simulink model "BicycleSimulation"  (R2020a)
settings: Solver=FixedStepAuto  StartTime=0.0  StopTime=inf  FixedStep=0.005  RelTol=1e-3  EnableMultiTasking=on
libraries: simulink x11
settings Model: NumberOfSteps=2  EnablePacing=on  Creator=Admin  LastModifiedBy=Robin Vogt
settings DataIOCC: ReturnWorkspaceOutputs=off
settings OptimizationCC: LifeSpan=inf
settings DebuggingCC: SFUnexpectedBacktrackingDiag=warning  SFNoUnconditionalDefaultTransitionDiag=warning  SFExecutionAtInitializationDiag=none  UnderSpecifiedDimensionMsg=warning  ArithmeticOperatorsInVariantConditions=warning
settings SFSimCC: SimUseLocalCustomCode=off  CustomCodeUndefinedFunction=UseInterfaceOnly
settings RTWCC: RTWUseLocalCustomCode=off
settings CodeAppCC: StateflowObjectComments=on
settings GRTTargetCC: TargetLangStandard=C89/C90 (ANSI)
settings ConfigComp: CovMetricSettings=dw  CovHtmlReporting=on  CovSaveCumulativeToWorkspaceVar=on  CovSaveSingleToWorkspaceVar=on  CovExternalEMLEnable=off

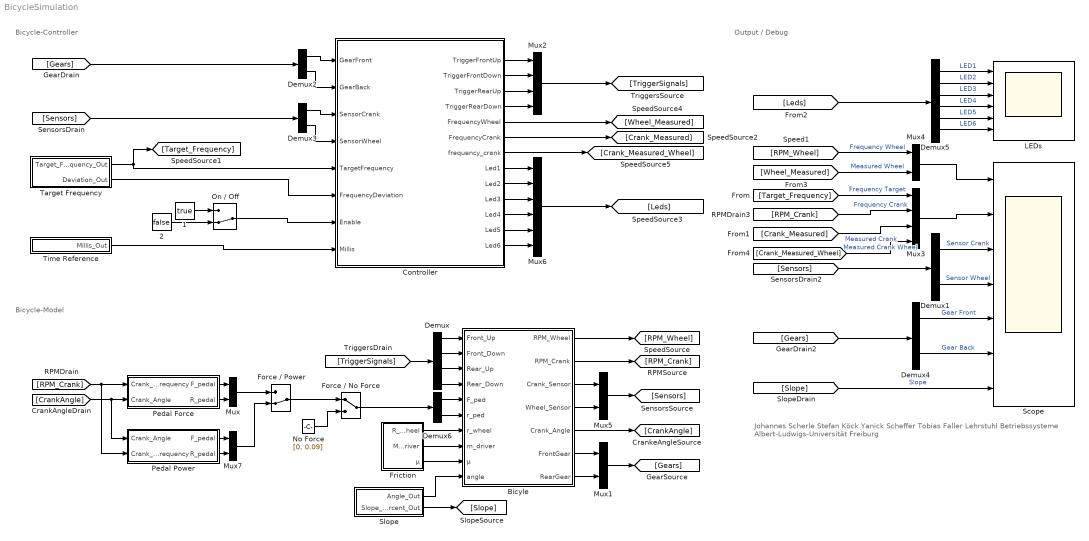
== system BicycleSimulation ==
  note: Bicycle-Model
  note: Johannes Scherle
      | Stefan Köck
      | Yanick Scheffer
      | Tobias Faller
      | Lehrstuhl Betriebssysteme
      | Albert-Ludwigs-Universität Freiburg
  note: Bicycle-Controller
  note: Output / Debug
  1 : Constant  Value=true  OutDataTypeStr=boolean
  2 : Constant  Value=false  OutDataTypeStr=boolean
  Bicyle : Subsystem
  Controller : Stateflow chart  TreatAsAtomicUnit=on  SystemSampleTime=0.005
      settings: PortSchema="{\"entries\":[{\"content\":{\"sides\":[{\"content\":{\"connectorIds\":[\"In1\",\"In2\",\"In3\",\"In4\",\"In5\",\"In6\",\"In7\",\"In8\"]},\"type\":\"ConnectorPlacement.EquallySpacedRectSide\",\"uuid\":\"1754ec92-7cce-411a-82a3-2fbca3fb4c28\"},{\"content\":{\"connectorIds\":[\"Out1\",\"Out2\",\"Out3\",\"Out4\",\"Out5\",\"Out6\",\"Out13\",\"Out7\",\"Out8\",\"Out9\",\"Out10\",\"Out11\",\"Out12\"],\"side\":\"RIGHT\"},\"type\":\"ConnectorPlacement.EquallySpacedRectSide\",\"uuid\":\"9c6a9c26-d673-4feb-91f9-24c7e2d76c42\"},{\"content\":{\"connectorIds\":[],\"side\":\"TOP\"},\"type\":\"ConnectorPlacement.EquallySpacedRectSide\",\"uuid\":\"a2f456d0-fed3-444f-af5e-51a24e4e3fa9\"}]},\"type\":\"ConnectorPlacement.EquallySpacedConnector\",\"uuid\":\"42155252-21b8-44f1-bf8e-e9314f1d83ec\"}],\"packageUris\":[\"http://schema.mathworks.com/mf0/Connector/19700101\"],\"version\":\"1.0\"}"
  Demux : Demux
  Demux{1..4,6} (5 alike) : Demux  Outputs=2
  Demux5 : Demux  Outputs=6
  Force / No Force : ManualSwitch
  Force / Power : ManualSwitch  CurrentSetting=0
  Friction : Subsystem
  LEDs : Scope  NumInputPorts=6
  Mux{,1,5,7} (4 alike) : Mux  Inputs=2
  Mux2 : Mux
  Mux3 : Mux  Inputs=Frequency Target,Frequency Crank,Measured Crank,Measured Crank Wheel
  Mux4 : Mux  Inputs=Frequency Wheel,Measured Wheel
  Mux6 : Mux  Inputs=6
  No Force : Constant  Value=[0, 0.09]  VectorParams1D=off  OutDataTypeStr=double
  On / Off : ManualSwitch  CurrentSetting=0
  Pedal Force : Subsystem
  Pedal Power : Subsystem
  Scope : Scope  NumInputPorts=7
  Slope : Subsystem
  Target Frequency : Subsystem
  Time Reference : Subsystem
  wires:
  Slope/1(Angle_Out) -> Bicyle/10(angle)
  Target Frequency/1(Target_Frequency_Out) -> Controller/5(TargetFrequency), [Target_Frequency]
  Target Frequency/2(Deviation_Out) -> Controller/6(FrequencyDeviation)
  Time Reference/1(Millis_Out) -> Controller/8(Millis)
  Bicyle/3(Crank_Sensor) -> Mux5/1
  Bicyle/4(Wheel_Sensor) -> Mux5/2
  Bicyle/6(FrontGear) -> Mux1/1
  Bicyle/7(RearGear) -> Mux1/2
  Controller/2(TriggerFrontDown) -> Mux2/2
  Controller/3(TriggerRearUp) -> Mux2/3
  Controller/1(TriggerFrontUp) -> Mux2/1
  Controller/4(TriggerRearDown) -> Mux2/4
  Demux/1 -> Bicyle/1(Front_Up)
  Demux/2 -> Bicyle/2(Front_Down)
  Demux/3 -> Bicyle/3(Rear_Up)
  Demux/4 -> Bicyle/4(Rear_Down)
  Mux2/1 -> [TriggerSignals]
  Demux4/1 -> Scope/5  "Gear Front"
  Demux4/2 -> Scope/6  "Gear Back"
  [TriggerSignals] -> Demux/1
  [Gears] -> Demux4/1
  Demux2/1 -> Controller/1(GearFront)
  Demux2/2 -> Controller/2(GearBack)
  Mux1/1 -> [Gears]
  Mux5/1 -> [Sensors]
  Friction/3(µ) -> Bicyle/9(µ)
  Friction/2(M_Driver) -> Bicyle/8(m_driver)
  Friction/1(R_Wheel) -> Bicyle/7(r_wheel)
  Demux1/2 -> Scope/4  "Sensor Wheel"
  [Sensors] -> Demux1/1
  Demux3/1 -> Controller/3(SensorCrank)
  Demux3/2 -> Controller/4(SensorWheel)
  Slope/2(Slope_Percent_Out) -> [Slope]
  [Slope] -> Scope/7  "Slope"
  Bicyle/5(Crank_Angle) -> [CrankAngle]
  [CrankAngle] -> Pedal Power/1(Crank_Angle), Pedal Force/2(Crank_Angle)
  Demux1/1 -> Scope/3  "Sensor Crank"
  Mux3/1 -> Scope/2
  Bicyle/2(RPM_Crank) -> [RPM_Crank]
  [RPM_Crank] -> Pedal Power/2(Crank_Frequency), Pedal Force/1(Crank_Frequency)
  [RPM_Crank] -> Mux3/2  "Frequency Crank"
  [Target_Frequency] -> Mux3/1  "Frequency Target"
  [Crank_Measured] -> Mux3/3  "Measured Crank"
  Controller/7(Led1) -> Mux6/1
  Controller/8(Led2) -> Mux6/2
  Controller/9(Led3) -> Mux6/3
  Controller/10(Led4) -> Mux6/4
  Controller/11(Led5) -> Mux6/5
  Controller/12(Led6) -> Mux6/6
  On / Off/1 -> Controller/7(Enable)
  1/1 -> On / Off/1
  2/1 -> On / Off/2
  Mux6/1 -> [Leds]
  [Sensors] -> Demux3/1
  [Gears] -> Demux2/1
  [Leds] -> Demux5/1
  Demux5/1 -> LEDs/1  "LED1"
  Demux5/2 -> LEDs/2  "LED2"
  Demux5/3 -> LEDs/3  "LED3"
  Demux5/4 -> LEDs/4  "LED4"
  Demux5/5 -> LEDs/5  "LED5"
  Demux5/6 -> LEDs/6  "LED6"
  Controller/5(FrequencyWheel) -> [Wheel_Measured]
  Bicyle/1(RPM_Wheel) -> [RPM_Wheel]
  Mux4/1 -> Scope/1
  [Wheel_Measured] -> Mux4/2  "Measured Wheel"
  [RPM_Wheel] -> Mux4/1  "Frequency Wheel"
  Mux/1 -> Force / Power/1
  Mux7/1 -> Force / Power/2
  Demux6/1 -> Bicyle/5(F_ped)
  Demux6/2 -> Bicyle/6(r_ped)
  Force / No Force/1 -> Demux6/1
  Force / Power/1 -> Force / No Force/1
  No Force/1 -> Force / No Force/2
  Pedal Force/1(F_pedal) -> Mux/1
  Pedal Force/2(R_pedal) -> Mux/2
  Pedal Power/1(F_pedal) -> Mux7/1
  Pedal Power/2(R_pedal) -> Mux7/2
  Controller/6(FrequencyCrank) -> [Crank_Measured]
  Controller/13(frequency_crank) -> [Crank_Measured_Wheel]
  [Crank_Measured_Wheel] -> Mux3/4  "Measured Crank Wheel"

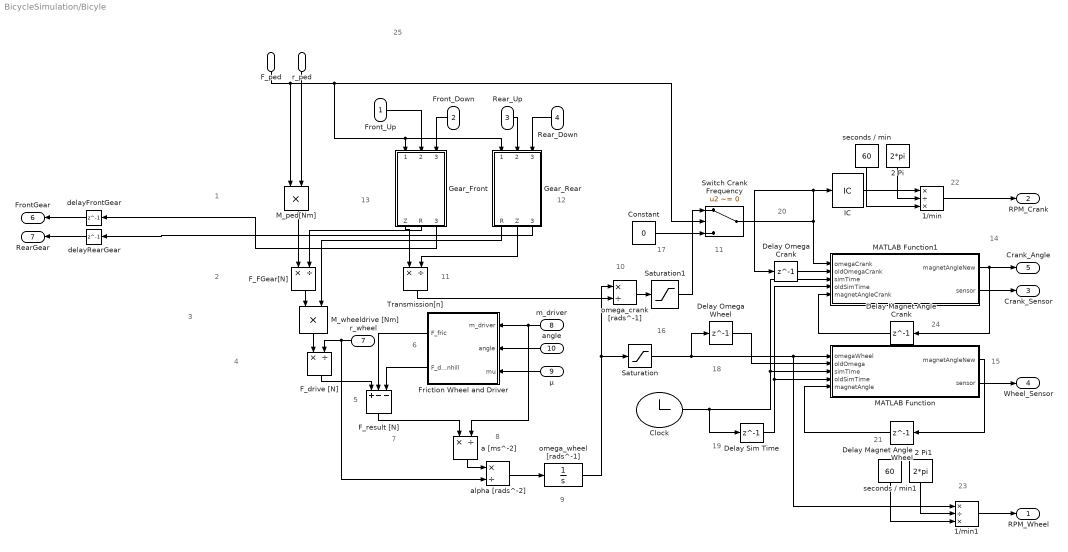
== system BicycleSimulation/Bicyle ==
  note: 1
  note: 2
  note: 3
  note: 4
  note: 5
  note: 6
  note: 7
  note: 8
  note: 9
  note: 10
  note: 11
  note: 11
  note: 12
  note: 13
  note: 14
  note: 15
  note: 16
  note: 17
  note: 18
  note: 19
  note: 20
  note: 21
  note: 22
  note: 23
  note: 24
  note: 25
  Front_Up : Inport
  Front_Down : Inport  Port=2
  Rear_Up : Inport  Port=3
  Rear_Down : Inport  Port=4
  F_ped : Inport  Port=5
  r_ped : Inport  Port=6
  r_wheel : Inport  Port=7
  m_driver : Inport  Port=8
  µ : Inport  Port=9
  angle : Inport  Port=10
  1/min : Product  Inputs=*/*  OutDataTypeStr=double
  1/min1 : Product  Inputs=*/*
  2 Pi : Constant  Value=2*pi
  2 Pi1 : Constant  Value=2*pi
  Clock : Clock
  Constant : Constant  Value=0
  Delay Omega Crank : Delay  DelayLength=1  InitialCondition=1
  Delay Omega Wheel : Delay  DelayLength=1  InitialCondition=0
  Delay Sim Time : Delay  DelayLength=1  InitialCondition=0
  "Delay Magnet Angle Crank " : Delay  DelayLength=1  InitialCondition=0
  Delay Magnet Angle Wheel : Delay  DelayLength=1  InitialCondition=0
  F_FGear[N] : Product  Inputs=*/
  F_drive [N] : Product  Inputs=*/
  F_result [N] : Sum  Inputs=+--
  Friction Wheel and Driver : Subsystem
  Gear_Front : Subsystem
  Gear_Rear : Subsystem
  IC : InitialCondition  Value=0
  MATLAB Function : MATLAB Function  TreatAsAtomicUnit=on
  MATLAB Function1 : MATLAB Function  TreatAsAtomicUnit=on
  M_ped[Nm] : Product
  M_wheeldrive [Nm] : Product
  Saturation : Saturate  UpperLimit=100  LowerLimit=0
  Saturation1 : Saturate  UpperLimit=18  LowerLimit=0
  Switch Crank Frequency : Switch  Criteria=u2 ~= 0
  Transmission[n] : Product  Inputs=*/
  a [ms^-2] : Product  Inputs=*/
  alpha [rads^-2] : Product  Inputs=*/
  delayFrontGear : Delay  DelayLength=1  InitialCondition=0
  delayRearGear : Delay  DelayLength=1  InitialCondition=0
  omega_crank [rads^-1] : Product  Inputs=*/
  omega_wheel [rads^-1] : Integrator  LimitOutput=on  UpperSaturationLimit=60  LowerSaturationLimit=0
  seconds / min : Constant  Value=60
  seconds / min1 : Constant  Value=60
  RPM_Wheel : Outport  VectorParamsAs1DForOutWhenUnconnected=off
  RPM_Crank : Outport  Port=2  VectorParamsAs1DForOutWhenUnconnected=off
  Crank_Sensor : Outport  Port=3  VectorParamsAs1DForOutWhenUnconnected=off
  Wheel_Sensor : Outport  Port=4  VectorParamsAs1DForOutWhenUnconnected=off
  Crank_Angle : Outport  Port=5  VectorParamsAs1DForOutWhenUnconnected=off
  FrontGear : Outport  Port=6  VectorParamsAs1DForOutWhenUnconnected=off
  RearGear : Outport  Port=7  VectorParamsAs1DForOutWhenUnconnected=off
  wires:
  Front_Up/1 -> Gear_Front/2(Trigger_Up)
  Rear_Up/1 -> Gear_Rear/2(Trigger_Up)
  Front_Down/1 -> Gear_Front/3(Trigger_Down)
  F_ped/1 -> Gear_Rear/1(F_ped), Gear_Front/1(F_ped), Switch Crank Frequency/2, M_ped[Nm]/1
  r_ped/1 -> M_ped[Nm]/2
  a [ms^-2]/1 -> alpha [rads^-2]/1
  M_ped[Nm]/1 -> F_FGear[N]/1
  M_wheeldrive [Nm]/1 -> F_drive [N]/1
  F_result [N]/1 -> a [ms^-2]/1
  Gear_Front/1(Z) -> Transmission[n]/1
  Gear_Front/2(R) -> F_FGear[N]/2
  F_FGear[N]/1 -> M_wheeldrive [Nm]/1
  Gear_Rear/1(R) -> M_wheeldrive [Nm]/2
  omega_crank [rads^-1]/1 -> Saturation1/1
  Friction Wheel and Driver/1(F_fric) -> F_result [N]/2
  Clock/1 -> Delay Sim Time/1, MATLAB Function/3(simTime), MATLAB Function1/3(simTime)
  Delay Omega Wheel/1 -> MATLAB Function/2(oldOmega)
  Delay Sim Time/1 -> MATLAB Function1/4(oldSimTime), MATLAB Function/4(oldSimTime)
  MATLAB Function/1(magnetAngleNew) -> Delay Magnet Angle Wheel/1
  Delay Magnet Angle Wheel/1 -> MATLAB Function/5(magnetAngle)
  MATLAB Function/2(sensor) -> Wheel_Sensor/1
  Rear_Down/1 -> Gear_Rear/3(Trigger_Down)
  r_wheel/1 -> F_drive [N]/2, alpha [rads^-2]/2
  F_drive [N]/1 -> F_result [N]/1
  Friction Wheel and Driver/2(F_downhill) -> F_result [N]/3
  m_driver/1 -> a [ms^-2]/2, Friction Wheel and Driver/1(m_driver)
  angle/1 -> Friction Wheel and Driver/2(angle)
  µ/1 -> Friction Wheel and Driver/3(mu)
  alpha [rads^-2]/1 -> omega_wheel [rads^-1]/1
  Gear_Rear/2(Z) -> Transmission[n]/2
  Delay Omega Crank/1 -> MATLAB Function1/2(oldOmegaCrank)
  MATLAB Function1/1(magnetAngleNew) -> "Delay Magnet Angle Crank "/1, Crank_Angle/1
  "Delay Magnet Angle Crank "/1 -> MATLAB Function1/5(magnetAngleCrank)
  MATLAB Function1/2(sensor) -> Crank_Sensor/1
  2 Pi/1 -> 1/min/2
  seconds / min/1 -> 1/min/3
  1/min/1 -> RPM_Crank/1
  Transmission[n]/1 -> omega_crank [rads^-1]/2
  Saturation/1 -> MATLAB Function/1(omegaWheel), 1/min1/1, Delay Omega Wheel/1
  2 Pi1/1 -> 1/min1/2
  seconds / min1/1 -> 1/min1/3
  1/min1/1 -> RPM_Wheel/1
  Switch Crank Frequency/1 -> Delay Omega Crank/1, IC/1, MATLAB Function1/1(omegaCrank)
  IC/1 -> 1/min/1
  omega_wheel [rads^-1]/1 -> omega_crank [rads^-1]/1, Saturation/1
  Gear_Rear/3(gearR) -> delayRearGear/1
  Gear_Front/3(gearF) -> delayFrontGear/1
  delayRearGear/1 -> RearGear/1
  delayFrontGear/1 -> FrontGear/1
  Saturation1/1 -> Switch Crank Frequency/1
  Constant/1 -> Switch Crank Frequency/3

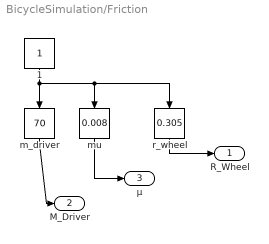
== system BicycleSimulation/Friction ==
  1 : Constant
  m_driver : simulink/Math Operations/Slider Gain  gain=70  low=0  high=150
  mu : simulink/Math Operations/Slider Gain  gain=0.008  low=0  high=0.1
  r_wheel : simulink/Math Operations/Slider Gain  gain=0.305  low=0  high=1
  R_Wheel : Outport  VectorParamsAs1DForOutWhenUnconnected=off
  M_Driver : Outport  Port=2  VectorParamsAs1DForOutWhenUnconnected=off
  µ : Outport  Port=3  VectorParamsAs1DForOutWhenUnconnected=off
  wires:
  m_driver/1 -> M_Driver/1
  r_wheel/1 -> R_Wheel/1
  1/1 -> m_driver/1, r_wheel/1, mu/1
  mu/1 -> µ/1

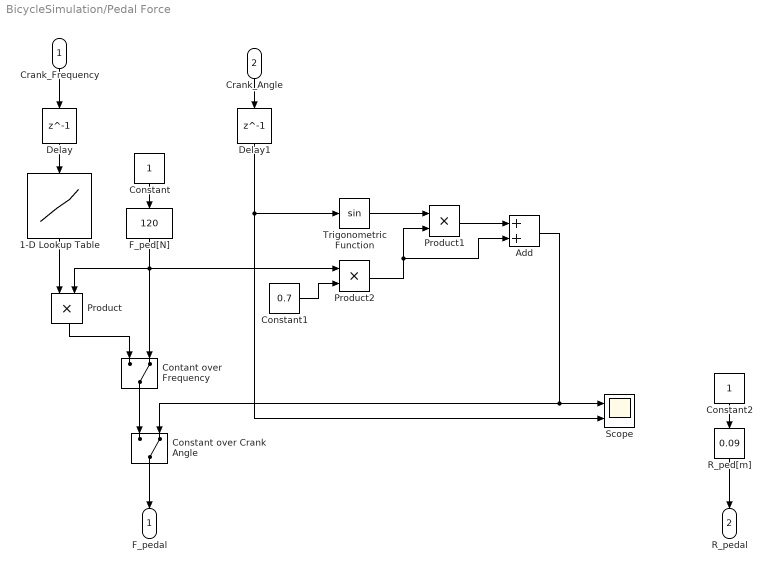
== system BicycleSimulation/Pedal Force ==
  Crank_Frequency : Inport
  Crank_Angle : Inport  Port=2
  1-D Lookup Table : Lookup_n-D  NumberOfTableDimensions=1  BreakpointsForDimension1=[0 10 20 30 40 50 60 70 80 90 100 110 120 130 140 150 160]  Table=[1 1 1 1 1 1 1 1 1 0.99 0.95 0.8 0.7 0.6 0.5 0.3 0]  RndMeth=Simplest  InputSameDT=on
  Add : Sum
  Constant : Constant
  Constant over Crank Angle : ManualSwitch  CurrentSetting=0
  Constant1 : Constant  Value=0.7
  Constant2 : Constant
  Contant over Frequency : ManualSwitch  CurrentSetting=0
  Delay : Delay  DelayLength=1
  Delay1 : Delay  DelayLength=1
  F_ped[N] : simulink/Math Operations/Slider Gain  gain=120  low=0  high=180
  Product : Product
  Product1 : Product
  Product2 : Product
  R_ped[m] : simulink/Math Operations/Slider Gain  gain=0.09  low=0  high=0.3
  Scope : Scope  NumInputPorts=2
  Trigonometric Function : Trigonometry
  F_pedal : Outport  VectorParamsAs1DForOutWhenUnconnected=off
  R_pedal : Outport  Port=2  VectorParamsAs1DForOutWhenUnconnected=off
  wires:
  R_ped[m]/1 -> R_pedal/1
  Constant/1 -> F_ped[N]/1
  F_ped[N]/1 -> Product/2, Contant over Frequency/2, Product2/1
  Product/1 -> Contant over Frequency/1
  1-D Lookup Table/1 -> Product/1
  Trigonometric Function/1 -> Product1/1
  Product2/1 -> Add/2, Product1/2
  Constant1/1 -> Product2/2
  Product1/1 -> Add/1
  Add/1 -> Scope/1, Constant over Crank Angle/2
  Constant over Crank Angle/1 -> F_pedal/1
  Contant over Frequency/1 -> Constant over Crank Angle/1
  Crank_Frequency/1 -> Delay/1
  Delay/1 -> 1-D Lookup Table/1
  Crank_Angle/1 -> Delay1/1
  Delay1/1 -> Trigonometric Function/1, Scope/2
  Constant2/1 -> R_ped[m]/1

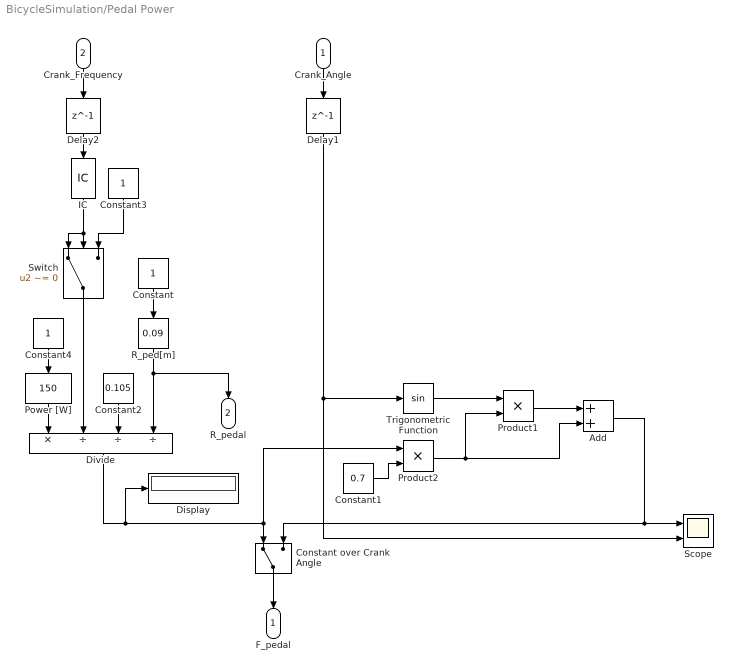
== system BicycleSimulation/Pedal Power ==
  Crank_Angle : Inport
  Crank_Frequency : Inport  Port=2
  Add : Sum
  Constant : Constant
  Constant over Crank Angle : ManualSwitch
  Constant1 : Constant  Value=0.7
  Constant2 : Constant  Value=0.105
  Constant3 : Constant
  Constant4 : Constant
  Delay1 : Delay  DelayLength=1
  Delay2 : Delay  DelayLength=1  InitialCondition=1
  Display : Display
  Divide : Product  Inputs=*///
  IC : InitialCondition
  Power [W] : simulink/Math Operations/Slider Gain  gain=150  low=0  high=200
  Product1 : Product
  Product2 : Product
  R_ped[m] : simulink/Math Operations/Slider Gain  gain=0.09  low=0  high=0.3
  Scope : Scope  NumInputPorts=2
  Switch : Switch  Criteria=u2 ~= 0
  Trigonometric Function : Trigonometry
  F_pedal : Outport  VectorParamsAs1DForOutWhenUnconnected=off
  R_pedal : Outport  Port=2  VectorParamsAs1DForOutWhenUnconnected=off
  wires:
  R_ped[m]/1 -> R_pedal/1, Divide/4
  Constant/1 -> R_ped[m]/1
  Power [W]/1 -> Divide/1
  Trigonometric Function/1 -> Product1/1
  Product2/1 -> Add/2, Product1/2
  Constant1/1 -> Product2/2
  Product1/1 -> Add/1
  Add/1 -> Scope/1, Constant over Crank Angle/2
  Constant over Crank Angle/1 -> F_pedal/1
  Constant2/1 -> Divide/3
  Divide/1 -> Constant over Crank Angle/1, Product2/1, Display/1
  Delay2/1 -> IC/1
  Crank_Frequency/1 -> Delay2/1
  Crank_Angle/1 -> Delay1/1
  Delay1/1 -> Scope/2, Trigonometric Function/1
  IC/1 -> Switch/1, Switch/2
  Constant3/1 -> Switch/3
  Switch/1 -> Divide/2
  Constant4/1 -> Power [W]/1

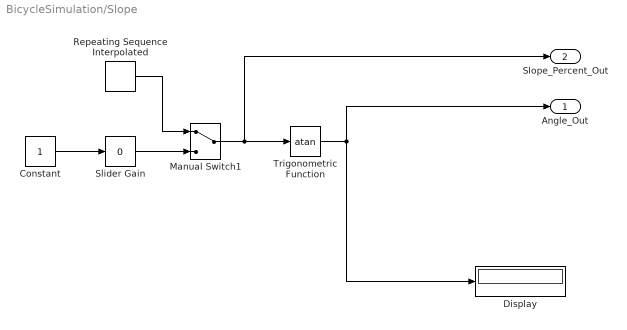
== system BicycleSimulation/Slope ==
  Constant : Constant
  Display : Display
  Manual Switch1 : ManualSwitch
  Repeating Sequence Interpolated : simulink/Sources/Repeating Sequence Interpolated  OutValues=[0 0.01 0.05 0.07 -0.05 -0.01 0].'  TimeValues=[0 2 4 6 8 10 12].'  LookUpMeth=Interpolation-Use End Values  tsamp=0.005  OutMin=[]  OutMax=[]  OutDataTypeStr=double  OutputDataTypeScalingMode=double  OutDataType=fixdt(0,8)  OutScaling=2^-10
  Slider Gain : simulink/Math Operations/Slider Gain  gain=0  low=-1  high=1
  Trigonometric Function : Trigonometry  Operator=atan
  Angle_Out : Outport  VectorParamsAs1DForOutWhenUnconnected=off
  Slope_Percent_Out : Outport  Port=2  VectorParamsAs1DForOutWhenUnconnected=off
  wires:
  Constant/1 -> Slider Gain/1
  Trigonometric Function/1 -> Angle_Out/1, Display/1
  Manual Switch1/1 -> Slope_Percent_Out/1, Trigonometric Function/1
  Slider Gain/1 -> Manual Switch1/2
  Repeating Sequence Interpolated/1 -> Manual Switch1/1

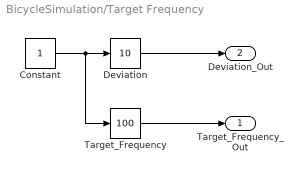
== system BicycleSimulation/Target Frequency ==
  Constant : Constant  OutDataTypeStr=double
  Deviation : simulink/Math Operations/Slider Gain  gain=10  low=0  high=20
  Target_Frequency : simulink/Math Operations/Slider Gain  gain=100  low=0  high=150
  Target_Frequency_Out : Outport  VectorParamsAs1DForOutWhenUnconnected=off
  Deviation_Out : Outport  Port=2  VectorParamsAs1DForOutWhenUnconnected=off
  wires:
  Constant/1 -> Deviation/1, Target_Frequency/1
  Target_Frequency/1 -> Target_Frequency_Out/1
  Deviation/1 -> Deviation_Out/1

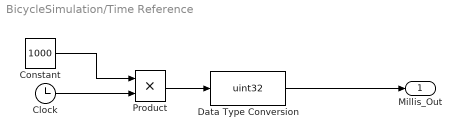
== system BicycleSimulation/Time Reference ==
  Clock : Clock
  Constant : Constant  Value=1000
  Data Type Conversion : DataTypeConversion  OutDataTypeStr=uint32
  Product : Product
  Millis_Out : Outport  SampleTime=0.005  VectorParamsAs1DForOutWhenUnconnected=off
  wires:
  Clock/1 -> Product/2
  Data Type Conversion/1 -> Millis_Out/1
  Product/1 -> Data Type Conversion/1
  Constant/1 -> Product/1

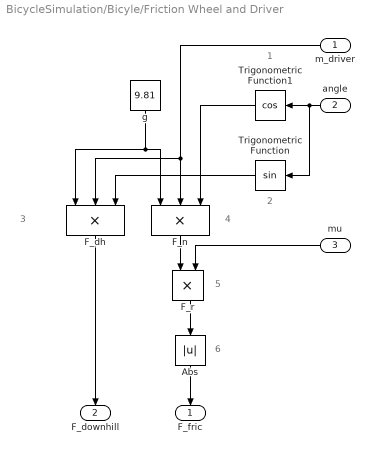
== system BicycleSimulation/Bicyle/Friction Wheel and Driver ==
  note: 1
  note: 2
  note: 3
  note: 4
  note: 5
  note: 6
  m_driver : Inport
  angle : Inport  Port=2
  mu : Inport  Port=3
  Abs : Abs
  F_dh : Product  Inputs=3
  F_n : Product  Inputs=3
  F_r : Product
  Trigonometric Function : Trigonometry
  Trigonometric Function1 : Trigonometry  Operator=cos
  g : Constant  Value=9.81
  F_fric : Outport  VectorParamsAs1DForOutWhenUnconnected=off
  F_downhill : Outport  Port=2  VectorParamsAs1DForOutWhenUnconnected=off
  wires:
  g/1 -> F_dh/1, F_n/1
  Abs/1 -> F_fric/1
  F_n/1 -> F_r/1
  F_r/1 -> Abs/1
  m_driver/1 -> F_dh/2, F_n/2
  Trigonometric Function1/1 -> F_n/3
  mu/1 -> F_r/2
  Trigonometric Function/1 -> F_dh/3
  F_dh/1 -> F_downhill/1
  angle/1 -> Trigonometric Function1/1, Trigonometric Function/1

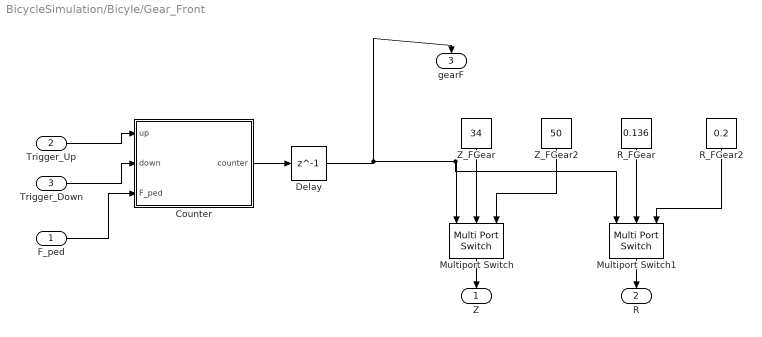
== system BicycleSimulation/Bicyle/Gear_Front ==
  F_ped : Inport
  Trigger_Up : Inport  Port=2
  Trigger_Down : Inport  Port=3
  Counter : Stateflow chart  TreatAsAtomicUnit=on
  Delay : Delay  DelayLength=1
  Multiport Switch : MultiPortSwitch  Inputs=2  DiagnosticForDefault=Warning
  Multiport Switch1 : MultiPortSwitch  Inputs=2  DiagnosticForDefault=Warning
  R_FGear : Constant  Value=0.136
  R_FGear2 : Constant  Value=0.2
  Z_FGear : Constant  Value=34
  Z_FGear2 : Constant  Value=50
  Z : Outport  VectorParamsAs1DForOutWhenUnconnected=off
  R : Outport  Port=2  VectorParamsAs1DForOutWhenUnconnected=off
  gearF : Outport  Port=3  VectorParamsAs1DForOutWhenUnconnected=off
  wires:
  Z_FGear2/1 -> Multiport Switch/3
  Z_FGear/1 -> Multiport Switch/2
  R_FGear/1 -> Multiport Switch1/2
  R_FGear2/1 -> Multiport Switch1/3
  Multiport Switch/1 -> Z/1
  Multiport Switch1/1 -> R/1
  Trigger_Down/1 -> Counter/2(down)
  Trigger_Up/1 -> Counter/1(up)
  F_ped/1 -> Counter/3(F_ped)
  Counter/1(counter) -> Delay/1
  Delay/1 -> Multiport Switch1/1, Multiport Switch/1, gearF/1

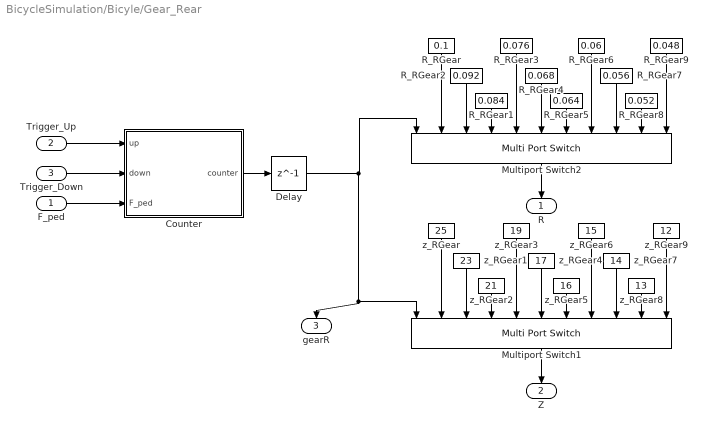
== system BicycleSimulation/Bicyle/Gear_Rear ==
  F_ped : Inport
  Trigger_Up : Inport  Port=2
  Trigger_Down : Inport  Port=3
  Counter : Stateflow chart  TreatAsAtomicUnit=on
  Delay : Delay  DelayLength=1
  Multiport Switch1 : MultiPortSwitch  Inputs=10  DiagnosticForDefault=Warning
  Multiport Switch2 : MultiPortSwitch  Inputs=10  DiagnosticForDefault=Warning
  R_RGear : Constant  Value=0.1
  R_RGear1 : Constant  Value=0.084
  R_RGear2 : Constant  Value=0.092
  R_RGear3 : Constant  Value=0.076
  R_RGear4 : Constant  Value=0.068
  R_RGear5 : Constant  Value=0.064
  R_RGear6 : Constant  Value=0.06
  R_RGear7 : Constant  Value=0.056
  R_RGear8 : Constant  Value=0.052
  R_RGear9 : Constant  Value=0.048
  z_RGear : Constant  Value=25
  z_RGear1 : Constant  Value=23
  z_RGear2 : Constant  Value=21
  z_RGear3 : Constant  Value=19
  z_RGear4 : Constant  Value=17
  z_RGear5 : Constant  Value=16
  z_RGear6 : Constant  Value=15
  z_RGear7 : Constant  Value=14
  z_RGear8 : Constant  Value=13
  z_RGear9 : Constant  Value=12
  R : Outport  VectorParamsAs1DForOutWhenUnconnected=off
  Z : Outport  Port=2  VectorParamsAs1DForOutWhenUnconnected=off
  gearR : Outport  Port=3  VectorParamsAs1DForOutWhenUnconnected=off
  wires:
  R_RGear2/1 -> Multiport Switch2/3
  R_RGear/1 -> Multiport Switch2/2
  Multiport Switch2/1 -> R/1
  Trigger_Down/1 -> Counter/2(down)
  Trigger_Up/1 -> Counter/1(up)
  R_RGear1/1 -> Multiport Switch2/4
  R_RGear3/1 -> Multiport Switch2/5
  R_RGear4/1 -> Multiport Switch2/6
  R_RGear5/1 -> Multiport Switch2/7
  R_RGear8/1 -> Multiport Switch2/10
  R_RGear7/1 -> Multiport Switch2/9
  R_RGear6/1 -> Multiport Switch2/8
  z_RGear1/1 -> Multiport Switch1/3
  z_RGear/1 -> Multiport Switch1/2
  Multiport Switch1/1 -> Z/1
  z_RGear2/1 -> Multiport Switch1/4
  z_RGear3/1 -> Multiport Switch1/5
  z_RGear4/1 -> Multiport Switch1/6
  z_RGear5/1 -> Multiport Switch1/7
  z_RGear8/1 -> Multiport Switch1/10
  z_RGear7/1 -> Multiport Switch1/9
  z_RGear6/1 -> Multiport Switch1/8
  z_RGear9/1 -> Multiport Switch1/11
  R_RGear9/1 -> Multiport Switch2/11
  F_ped/1 -> Counter/3(F_ped)
  Counter/1(counter) -> Delay/1
  Delay/1 -> Multiport Switch1/1, gearR/1, Multiport Switch2/1

== stateflow chart BicycleSimulation/Controller ==
  settings: updateMethod=DISCRETE  sampleTime=0.005
  state Enabled
    state Calculations/ [parallel]
      gear = uint8(6)*(GearFront - uint8(1)) + GearBack;
      settings: executionOrder=1
      state Wheel_Speed_Calculation [parallel]
        settings: executionOrder=1
        state Signal
        Enabled.Calculations.Wheel_Speed_Calculation.Signal -> Enabled.Calculations.Wheel_Speed_Calculation.Signal [order 1] : [Millis >= start_time + time_interval && hasChangedTo(SensorWheel, 0)]/{
            | FrequencyWheel = double(6e4*(sensor_count+1)/(time_interval*16));
            | sensor_count = 0;
            | start_time = Millis;
            | }
        (default) -> Enabled.Calculations.Wheel_Speed_Calculation.Signal
        Enabled.Calculations.Wheel_Speed_Calculation.Signal -> Enabled.Calculations.Wheel_Speed_Calculation.Signal [order 2] : [ Millis < start_time + time_interval && hasChangedTo(SensorWheel, 0)]/{
            | sensor_count = sensor_count +  1;
            | }
      state Force [parallel]
        settings: executionOrder=3
        state Signal/
          en: start_time = Millis;
        Enabled.Calculations.Force.Signal -> Enabled.Calculations.Force.Signal [order 1] : [Millis < start_time + no_force_interval && hasChangedTo(SensorCrank, 0)]/
            | {force = true;}
        (default) -> Enabled.Calculations.Force.Signal
        Enabled.Calculations.Force.Signal -> Enabled.Calculations.Force.Signal [order 2] : [Millis >= start_time + no_force_interval]/{force = false;}
      state Crank_Speed_Calculation [parallel]
        settings: executionOrder=2
        state Signal/
          en: start_time = Millis;
        (default) -> Enabled.Calculations.Crank_Speed_Calculation.Signal
        Enabled.Calculations.Crank_Speed_Calculation.Signal -> Enabled.Calculations.Crank_Speed_Calculation.Signal : [hasChangedTo(SensorCrank, 0)]/{
            | period = Millis-start_time;
            | no_force_interval = 2*period;
            | FrequencyCrank = double(6e4/period);
            | }
    state Shifting [parallel]
      settings: executionOrder=2
      state Shift_gears/
        target_gear_front = idivide(target_gear - uint8(1),  uint8(8)) + uint8(1);
        target_gear_back = target_gear - uint8(6)*(target_gear_front - uint8(1));
        state Rear
          state Up
          state Timer/
            en:
            TriggerRearDown = false;
            TriggerRearUp = false;
            mutex = false;
            start_time = Millis;
            ex:
            mutex = true;
          state Down
          Enabled.Shifting.Shift_gears.Rear.Up -> (junction 210)
          (junction 204) -> Enabled.Shifting.Shift_gears.Rear.Up [order 2] : [GearBack < target_gear_back]/{TriggerRearUp = true;}
          (default) -> Enabled.Shifting.Shift_gears.Rear.Timer
          (junction 210) -> Enabled.Shifting.Shift_gears.Rear.Timer : [Millis >= start_time + uint32(50)]/
              | {servo_timer_rear = Millis;}
          Enabled.Shifting.Shift_gears.Rear.Timer -> (junction 204) : [Millis - servo_timer_rear > uint32(100)]
          Enabled.Shifting.Shift_gears.Rear.Down -> (junction 210)
          (junction 204) -> Enabled.Shifting.Shift_gears.Rear.Down [order 1] : [GearBack > target_gear_back]/{TriggerRearDown = true;}
        state Front
          state Up
          state Timer/
            en:
            TriggerFrontDown = false;
            TriggerFrontUp = false;
            mutex = false;
            start_time = Millis;
            ex:
            mutex = true;
          state Down
          Enabled.Shifting.Shift_gears.Front.Up -> (junction 194)
          (default) -> Enabled.Shifting.Shift_gears.Front.Timer
          (junction 187) -> Enabled.Shifting.Shift_gears.Front.Up [order 1] : [GearFront < target_gear_front]/{TriggerFrontUp = true;}
          Enabled.Shifting.Shift_gears.Front.Timer -> (junction 187) : [Millis - servo_timer_front > 500]
          (junction 194) -> Enabled.Shifting.Shift_gears.Front.Timer : [Millis >= start_time + 600]/
              | {servo_timer_front = Millis;}
          (junction 187) -> Enabled.Shifting.Shift_gears.Front.Down [order 2] : [GearFront > target_gear_front]/{TriggerFrontDown = true;}
          Enabled.Shifting.Shift_gears.Front.Down -> (junction 194)
        Rear -> Front : [GearFront ~= target_gear_front && GearBack > 2 && GearBack < 9]
        (default) -> Rear
        Front -> Rear : [GearFront == target_gear_front]
      state Shifting_decision/
        en:
        translation = translations(gear);
        du:
        frequency_crank = FrequencyWheel/translation;
        state Constant_speed
        state Timer/
          en:
          start_time = Millis;
        state Find_target_gear/
          en:
          lower_bound = bounds(1, index);
          upper_bound = bounds(2, index);
        (default) -> Constant_speed
        Constant_speed -> Enabled.Shifting.Shifting_decision.Timer : [frequency_crank > TargetFrequency + FrequencyDeviation || frequency_crank < TargetFrequency - FrequencyDeviation]
        Enabled.Shifting.Shifting_decision.Timer -> Constant_speed [order 2] : [frequency_crank > TargetFrequency - FrequencyDeviation && frequency_crank < TargetFrequency + FrequencyDeviation]
        (junction 233) -> Constant_speed
        Enabled.Shifting.Shifting_decision.Timer -> Find_target_gear [order 1] : [Millis >= start_time + buffer]/
            | {target_translation = FrequencyWheel/TargetFrequency;
            | index = gear;}
        Find_target_gear -> Find_target_gear [order 3] : [target_translation < lower_bound]/
            | {index = index - 1;}
        Find_target_gear -> Find_target_gear [order 2] : [target_translation > upper_bound]/
            | {index = index + 1;}
        Find_target_gear -> (junction 234) [order 1] : [target_translation <= upper_bound && target_translation >= lower_bound]/
            | {target_gear = index;}
        (junction 234) -> (junction 233)
      state Wait_for_Measurement
      note: need to guard that transition with a mutex
      (default) -> Wait_for_Measurement
      Shifting_decision -> Shift_gears : [gear ~= target_gear && force]
      Wait_for_Measurement -> Shifting_decision : [hasChanged(GearFront) && hasChanged(GearBack)]/
          | {gear = uint8(6)*(GearFront - uint8(1)) + GearBack;}
      Shift_gears -> Shifting_decision : [~mutex && (~force || gear == target_gear)]
  state Disabled
  (default) -> Disabled
  Enabled -> Disabled : [~Enable]
  Disabled -> Enabled : [Enable]
  data: start_time local uint32 =uint32(0); sensor_count local uint32 =uint32(0); time_interval local uint32 =uint32(500); start_time local uint32 =uint32(0); start_time local uint32 =uint32(0); period local uint32; no_force_interval local uint32 =uint32(10000); start_time local; start_time local uint32; servo_timer_front local uint32 =uint32(0); servo_timer_rear local uint32 =uint32(0); target_translation local double; upper_bound local double; lower_bound local double; buffer constant uint32 =uint32(1e3); start_time local uint32 =uint32(0); upper_bounds constant double size=[2 8] =[1.42 1.55 1.705 1.895 2.065 2.2 2.35 2.53; 2.525 2.785 2.035 3.23 3.42 3.71 4.01 0]; lower_bounds constant double size=[2 8] =[0 1.42 1.55 1.705 1.895 2.065 2.2 2.35; 2.325 2.525 2.785 2.035 3.23 3.42 3.71 4.01]; translation local double; translations constant double size=[1 16] =[1.36 1.48 1.62 1.79 2.00 2.13 2.27 2.43 2.38 2.63 2.94 3.13 3.33 3.57 3.85 4.17]; index local uint8; bounds constant double size=[2 16] =[0 1.42 1.55 1.705 1.895 2.065 2.2 2.35 2.325 2.525 2.785 2.035 3.23 3.42 3.71 4.01; 1.42 1.55 1.705 1.895 2.065 2.2 2.35 2.53 2.525 2.785 2.035 3.23 3.42 3.71 4.01 100]; mutex local boolean =false; GearFront input uint8; GearBack input uint8; SensorCrank input boolean; SensorWheel input boolean; TargetFrequency input double; TriggerFrontUp output boolean =false; TriggerFrontDown output boolean =false; TriggerRearUp output boolean =false; TriggerRearDown output boolean =false; FrequencyDeviation input double; Enable input boolean; FrequencyWheel output double =0.0; FrequencyCrank output double =0.0; Millis input uint32; Led1 output boolean =false; Led2 output boolean =false; Led3 output boolean =false; Led4 output boolean =false; Led5 output boolean =false; Led6 output boolean =false; force local boolean =true; target_gear_front local uint8 =uint8(1); target_gear_back local uint8 =uint8(1); gear local uint8; target_gear local uint8 =uint8(1); frequency_crank output double =0.0

== matlab function BicycleSimulation/Bicyle/MATLAB Function ==
  data: omegaWheel input; oldOmega input; magnetAngleNew output; simTime input; oldSimTime input; sensor output; magnetAngle input
function [magnetAngleNew, sensor]  = genSensorSignal(omegaWheel, oldOmega, ...
                                                     simTime, oldSimTime, ...
                                                     magnetAngle)

% Calculate the mean omega in between the last two simulation steps.
meanOmega = (omegaWheel + oldOmega) / 2;

% Calculate the time between the two simulation steps.
timeLength = simTime - oldSimTime;

% Calculate the advance of the magnet between the last two simulation steps
% and add it to the angle of the magnet.
magnetAdvance = meanOmega * timeLength;
magnetAngleNew = magnetAngle + magnetAdvance;
magnetAngleNew = mod(magnetAngleNew, pi / 8); % signal 16 times per round

% Generate a peak when one round is completed
if magnetAngleNew < magnetAngle
    sensor = false;
else
    sensor = true;
end

== stateflow chart BicycleSimulation/Bicyle/Gear_Front/Counter ==
  state counter
  (junction 7) -> counter : [counter < 2] /
      | {counter = counter + 1;}
  counter -> (junction 7) [order 2] : [hasChangedTo(up, true) && F_ped > 0]
  (default) -> counter : /{counter = uint8(1);}
  counter -> (junction 11) [order 1] : [hasChangedTo(down, true) &&F_ped > 0]
  (junction 11) -> counter : [counter > 1 ]/
      | {counter = counter - 1;}
  data: up input boolean size=1; down input boolean size=1; counter output uint8 size=1; F_ped input double size=1

== stateflow chart BicycleSimulation/Bicyle/Gear_Rear/Counter ==
  state counter
  (junction 7) -> counter : [counter < 10] /
      | {counter = counter + 1;}
  counter -> (junction 7) [order 2] : [hasChangedTo(up, true) && F_ped > 0]
  (default) -> counter : /{counter = uint8(1);}
  counter -> (junction 11) [order 1] : [hasChangedTo(down, true) && F_ped > 0]
  (junction 11) -> counter : [counter > 1 ]/
      | {counter = counter - 1;}
  data: up input boolean size=1; down input boolean size=1; counter output uint8 size=1; F_ped input double size=1

== matlab function BicycleSimulation/Bicyle/MATLAB Function1 ==
  data: omegaCrank input; oldOmegaCrank input; magnetAngleNew output; simTime input; oldSimTime input; sensor output; magnetAngleCrank input
function [magnetAngleNew, sensor]  = genSensorSignal(omegaCrank, oldOmegaCrank, ...
                                                     simTime, oldSimTime, ...
                                                     magnetAngleCrank)

% Calculate the mean omega in between the last two simulation steps.
meanOmega = (omegaCrank + oldOmegaCrank) / 2;

% Calculate the time between the two simulation steps.
timeLength = simTime - oldSimTime;

% Calculate the advance of the magnet between the last two simulation steps
% and add it to the angle of the magnet.
magnetAdvance = meanOmega * timeLength;
magnetAngleNew = magnetAngleCrank + magnetAdvance;
magnetAngleNew = mod(magnetAngleNew, 2 * pi);

% Generate a peak when one round is completed
if magnetAngleNew < magnetAngleCrank
    sensor = false;
else
    sensor = true;
end
